simulink model "ThermoDynamicsFMU"  (R2023b)
settings: Solver=FixedStepAuto  StartTime=0.0  StopTime=200  FixedStep=1  RelTol=1e-3
undefined symbols (not defined in the file or in its folder): A, A_amb, Cp, delta_H, h, h_amb, rho, t_step, Vol
settings Model: Creator=20181234  LastModifiedBy=20181234

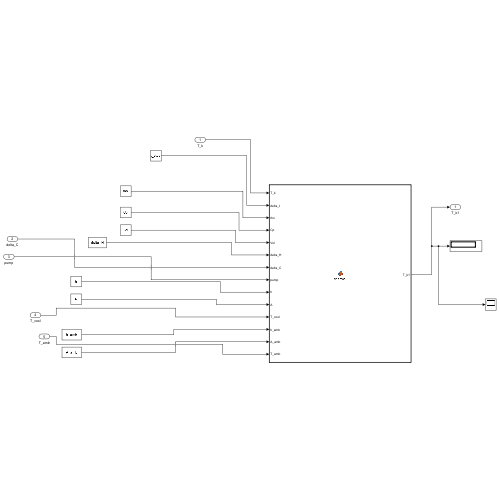
[thumbnail: Simulink's stored preview of the top-level diagram]
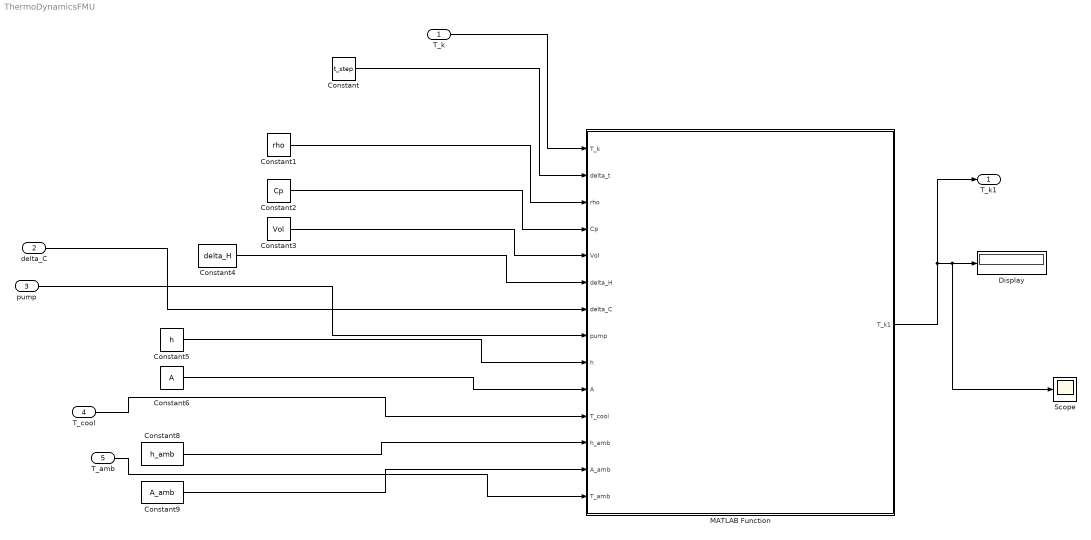
== system ThermoDynamicsFMU ==
  T_k : Inport
  delta_C : Inport  Port=2
  pump : Inport  Port=3
  T_cool : Inport  Port=4
  T_amb : Inport  Port=5
  Constant : Constant  Value=t_step
  Constant1 : Constant  Value=rho
  Constant2 : Constant  Value=Cp
  Constant3 : Constant  Value=Vol
  Constant4 : Constant  Value=delta_H
  Constant5 : Constant  Value=h
  Constant6 : Constant  Value=A
  Constant8 : Constant  Value=h_amb
  Constant9 : Constant  Value=A_amb
  Display : Display
  MATLAB Function : MATLAB Function  TreatAsAtomicUnit=on
  Scope : Scope
  T_k1 : Outport
  wires:
  T_amb/1 -> MATLAB Function/14(T_amb)
  T_cool/1 -> MATLAB Function/11(T_cool)
  Constant8/1 -> MATLAB Function/12(h_amb)
  Constant1/1 -> MATLAB Function/3(rho)
  Constant5/1 -> MATLAB Function/9(h)
  Constant/1 -> MATLAB Function/2(delta_t)
  Constant3/1 -> MATLAB Function/5(Vol)
  Constant2/1 -> MATLAB Function/4(Cp)
  Constant9/1 -> MATLAB Function/13(A_amb)
  T_k/1 -> MATLAB Function/1(T_k)
  pump/1 -> MATLAB Function/8(pump)
  delta_C/1 -> MATLAB Function/7(delta_C)
  MATLAB Function/1(T_k1) -> T_k1/1, Scope/1, Display/1
  Constant6/1 -> MATLAB Function/10(A)
  Constant4/1 -> MATLAB Function/6(delta_H)

== matlab function ThermoDynamicsFMU/MATLAB Function ==
  data: T_k input; T_k1 output; delta_t input; rho input; Cp input; Vol input; delta_H input; delta_C input; pump input; h input; A input; T_cool input; h_amb input; A_amb input; T_amb input
function T_k1 = thermo(T_k,delta_t, rho, Cp, Vol, delta_H, delta_C, pump, h, A, T_cool,h_amb, A_amb, T_amb)


factor = delta_t / (rho * Cp * (Vol/1000));
T_k1 = factor * (delta_H * delta_C*Vol - pump * h *60/1000 * A * (T_k - T_cool)-h_amb *60/1000 * A_amb * (T_k - T_amb)) + T_k;
